simulink model "AEB_System"  (R2023a)
settings: Solver=FixedStepAuto  StartTime=0.0  StopTime=10.0  FixedStep=1  RelTol=1e-3
values from neighbouring files (symbols this model uses):
  AEB_Brake_Apply = 1.0    [AEB_Data.sldd]
  AEB_Warning = 1.0    [AEB_Data.sldd]
  Friction = 0.7    [AEB_Data.sldd]
  Gravity = 9.81    [AEB_Data.sldd]
  Growth_Time_Dec = 0.1    [AEB_Data.sldd]
  L_Limit = -1.1    [AEB_Data.sldd]
  Min_Dis_Stop_Veh = 2.0    [AEB_Data.sldd]
  No_Warning = 0.0    [AEB_Data.sldd]
  On_Value = 1.0    [AEB_Data.sldd]
  Out_Rang = 300.0    [AEB_Data.sldd]
  R_Limit = 1.1    [AEB_Data.sldd]
  Reac_Time = 1.0    [AEB_Data.sldd]
settings Model: DataDictionary=AEB_Data.sldd  Creator=songi  LastModifiedBy=songi
settings DebuggingCC: ParameterPrecisionLossMsg=none  UnitsInconsistencyMsg=none

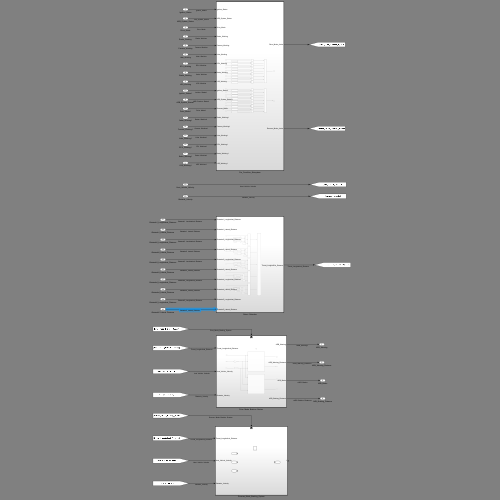
[thumbnail: Simulink's stored preview of the top-level diagram]
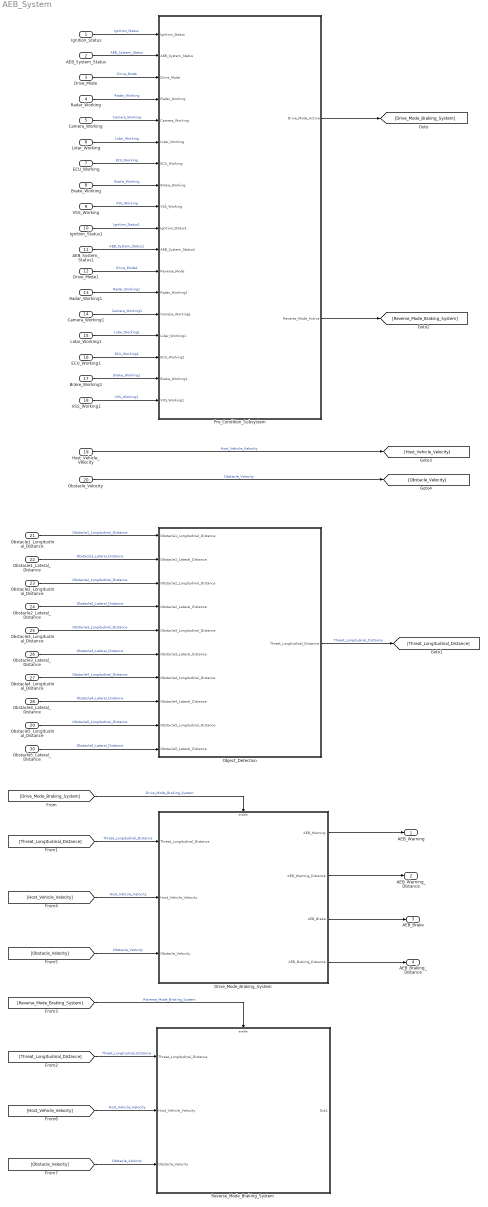
== system AEB_System ==
  Ignition_Status : Inport
  AEB_System_Status : Inport  Port=2
  Drive_Mode : Inport  Port=3
  Radar_Working : Inport  Port=4
  Camera_Working : Inport  Port=5
  Lidar_Working : Inport  Port=6
  ECU_Working : Inport  Port=7
  Brake_Working : Inport  Port=8
  VSS_Working : Inport  Port=9
  Ignition_Status1 : Inport  Port=10
  AEB_System_Status1 : Inport  Port=11
  Drive_Mode1 : Inport  Port=12
  Radar_Working1 : Inport  Port=13
  Camera_Working1 : Inport  Port=14
  Lidar_Working1 : Inport  Port=15
  ECU_Working1 : Inport  Port=16
  Brake_Working1 : Inport  Port=17
  VSS_Working1 : Inport  Port=18
  Host_Vehicle_Velocity : Inport  Port=19
  Obstacle_Velocity : Inport  Port=20
  Obstacle1_Longitudinal_Distance : Inport  Port=21
  Obstacle1_Lateral_Distance : Inport  Port=22
  Obstacle2_Longitudinal_Distance : Inport  Port=23
  Obstacle2_Lateral_Distance : Inport  Port=24
  Obstacle3_Longitudinal_Distance : Inport  Port=25
  Obstacle3_Lateral_Distance : Inport  Port=26
  Obstacle4_Longitudinal_Distance : Inport  Port=27
  Obstacle4_Lateral_Distance : Inport  Port=28
  Obstacle5_Longitudinal_Distance : Inport  Port=29
  Obstacle5_Lateral_Distance : Inport  Port=30
  Drive_Mode_Braking_System : Subsystem  TreatAsAtomicUnit=on
  Object_Detection : Subsystem  TreatAsAtomicUnit=on
  Pre_Condition_Subsystem : Subsystem  TreatAsAtomicUnit=on
  Reverse_Mode_Braking_System : Subsystem  TreatAsAtomicUnit=on
  AEB_Warning : Outport
  AEB_Warning_Distance : Outport  Port=2
  AEB_Brake : Outport  Port=3
  AEB_Braking_Distance : Outport  Port=4
  wires:
  Ignition_Status/1 -> Pre_Condition_Subsystem/1(Ignition_Status)  "Ignition_Status"
  AEB_System_Status/1 -> Pre_Condition_Subsystem/2(AEB_System_Status)  "AEB_System_Status"
  Drive_Mode/1 -> Pre_Condition_Subsystem/3(Drive_Mode)  "Drive_Mode"
  Radar_Working/1 -> Pre_Condition_Subsystem/4(Radar_Working)  "Radar_Working"
  Camera_Working/1 -> Pre_Condition_Subsystem/5(Camera_Working)  "Camera_Working"
  Lidar_Working/1 -> Pre_Condition_Subsystem/6(Lidar_Working)  "Lidar_Working"
  ECU_Working/1 -> Pre_Condition_Subsystem/7(ECU_Working)  "ECU_Working"
  Brake_Working/1 -> Pre_Condition_Subsystem/8(Brake_Working)  "Brake_Working"
  VSS_Working/1 -> Pre_Condition_Subsystem/9(VSS_Working)  "VSS_Working"
  Obstacle2_Longitudinal_Distance/1 -> Object_Detection/3(Obstacle2_Longitudinal_Distance)  "Obstacle2_Longitudinal_Distance"
  Obstacle2_Lateral_Distance/1 -> Object_Detection/4(Obstacle2_Lateral_Distance)  "Obstacle2_Lateral_Distance"
  Obstacle3_Longitudinal_Distance/1 -> Object_Detection/5(Obstacle3_Longitudinal_Distance)  "Obstacle3_Longitudinal_Distance"
  Obstacle3_Lateral_Distance/1 -> Object_Detection/6(Obstacle3_Lateral_Distance)  "Obstacle3_Lateral_Distance"
  Obstacle4_Longitudinal_Distance/1 -> Object_Detection/7(Obstacle4_Longitudinal_Distance)  "Obstacle4_Longitudinal_Distance"
  Obstacle4_Lateral_Distance/1 -> Object_Detection/8(Obstacle4_Lateral_Distance)  "Obstacle4_Lateral_Distance"
  Obstacle5_Longitudinal_Distance/1 -> Object_Detection/9(Obstacle5_Longitudinal_Distance)  "Obstacle5_Longitudinal_Distance"
  Obstacle5_Lateral_Distance/1 -> Object_Detection/10(Obstacle5_Lateral_Distance)  "Obstacle5_Lateral_Distance"
  Pre_Condition_Subsystem/1(Drive_Mode_Active) -> [Drive_Mode_Braking_System]
  Pre_Condition_Subsystem/2(Reverse_Mode_Active) -> [Reverse_Mode_Braking_System]
  Ignition_Status1/1 -> Pre_Condition_Subsystem/10(Ignition_Status1)  "Ignition_Status1"
  VSS_Working1/1 -> Pre_Condition_Subsystem/18(VSS_Working1)  "VSS_Working1"
  AEB_System_Status1/1 -> Pre_Condition_Subsystem/11(AEB_System_Status1)  "AEB_System_Status1"
  Drive_Mode1/1 -> Pre_Condition_Subsystem/12(Reverse_Mode)  "Drive_Mode1"
  Radar_Working1/1 -> Pre_Condition_Subsystem/13(Radar_Working1)  "Radar_Working1"
  Camera_Working1/1 -> Pre_Condition_Subsystem/14(Camera_Working1)  "Camera_Working1"
  ECU_Working1/1 -> Pre_Condition_Subsystem/16(ECU_Working1)  "ECU_Working1"
  Lidar_Working1/1 -> Pre_Condition_Subsystem/15(Lidar_Working1)  "Lidar_Working1"
  Brake_Working1/1 -> Pre_Condition_Subsystem/17(Brake_Working1)  "Brake_Working1"
  Object_Detection/1(Threat_Longitudinal_Distance) -> [Threat_Longitudinal_Distance]  "Threat_Longitudinal_Distance"
  Host_Vehicle_Velocity/1 -> [Host_Vehicle_Velocity]  "Host_Vehicle_Velocity"
  Obstacle1_Longitudinal_Distance/1 -> Object_Detection/1(Obstacle1_Longitudinal_Distance)  "Obstacle1_Longitudinal_Distance"
  Obstacle1_Lateral_Distance/1 -> Object_Detection/2(Obstacle1_Lateral_Distance)  "Obstacle1_Lateral_Distance"
  Obstacle_Velocity/1 -> [Obstacle_Velocity]  "Obstacle_Velocity"
  [Threat_Longitudinal_Distance] -> Drive_Mode_Braking_System/1(Threat_Longitudinal_Distance)  "Threat_Longitudinal_Distance"
  [Obstacle_Velocity] -> Drive_Mode_Braking_System/3(Obstacle_Velocity)  "Obstacle_Velocity"
  [Reverse_Mode_Braking_System] -> Reverse_Mode_Braking_System/Enable  "Reverse_Mode_Braking_System"
  [Obstacle_Velocity] -> Reverse_Mode_Braking_System/3(Obstacle_Velocity)  "Obstacle_Velocity"
  [Threat_Longitudinal_Distance] -> Reverse_Mode_Braking_System/1(Threat_Longitudinal_Distance)  "Threat_Longitudinal_Distance"
  [Drive_Mode_Braking_System] -> Drive_Mode_Braking_System/Enable  "Drive_Mode_Braking_System"
  [Host_Vehicle_Velocity] -> Reverse_Mode_Braking_System/2(Host_Vehicle_Velocity)  "Host_Vehicle_Velocity"
  Drive_Mode_Braking_System/1(AEB_Warning) -> AEB_Warning/1
  Drive_Mode_Braking_System/2(AEB_Warning_Distance) -> AEB_Warning_Distance/1
  Drive_Mode_Braking_System/3(AEB_Brake) -> AEB_Brake/1
  Drive_Mode_Braking_System/4(AEB_Braking_Distance) -> AEB_Braking_Distance/1
  [Host_Vehicle_Velocity] -> Drive_Mode_Braking_System/2(Host_Vehicle_Velocity)  "Host_Vehicle_Velocity"

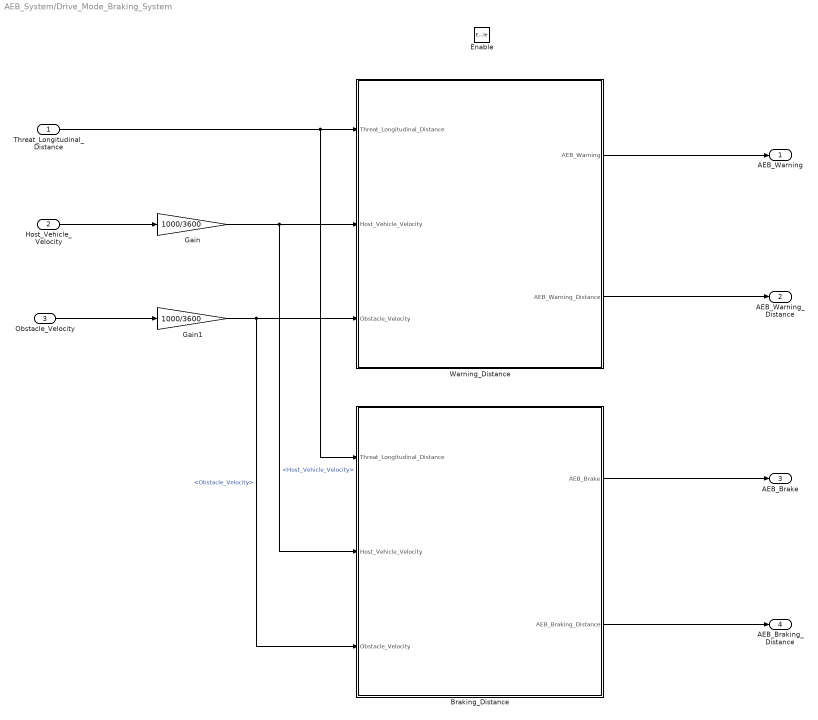
== system AEB_System/Drive_Mode_Braking_System ==
  Threat_Longitudinal_Distance : Inport
  Host_Vehicle_Velocity : Inport  Port=2
  Obstacle_Velocity : Inport  Port=3
  Enable : EnablePort
  Braking_Distance : Subsystem  TreatAsAtomicUnit=on
  Gain : Gain  Gain=1000/3600  OutDataTypeStr=half
  Gain1 : Gain  Gain=1000/3600  OutDataTypeStr=half
  Warning_Distance : Subsystem  TreatAsAtomicUnit=on
  AEB_Warning : Outport
  AEB_Warning_Distance : Outport  Port=2
  AEB_Brake : Outport  Port=3
  AEB_Braking_Distance : Outport  Port=4
  wires:
  Threat_Longitudinal_Distance/1 -> Braking_Distance/1(Threat_Longitudinal_Distance), Warning_Distance/1(Threat_Longitudinal_Distance)
  Warning_Distance/1(AEB_Warning) -> AEB_Warning/1
  Warning_Distance/2(AEB_Warning_Distance) -> AEB_Warning_Distance/1
  Braking_Distance/1(AEB_Brake) -> AEB_Brake/1
  Braking_Distance/2(AEB_Braking_Distance) -> AEB_Braking_Distance/1
  Obstacle_Velocity/1 -> Gain1/1
  Gain1/1 -> Braking_Distance/3(Obstacle_Velocity), Warning_Distance/3(Obstacle_Velocity)  "<Obstacle_Velocity>"
  Host_Vehicle_Velocity/1 -> Gain/1
  Gain/1 -> Braking_Distance/2(Host_Vehicle_Velocity), Warning_Distance/2(Host_Vehicle_Velocity)  "<Host_Vehicle_Velocity>"

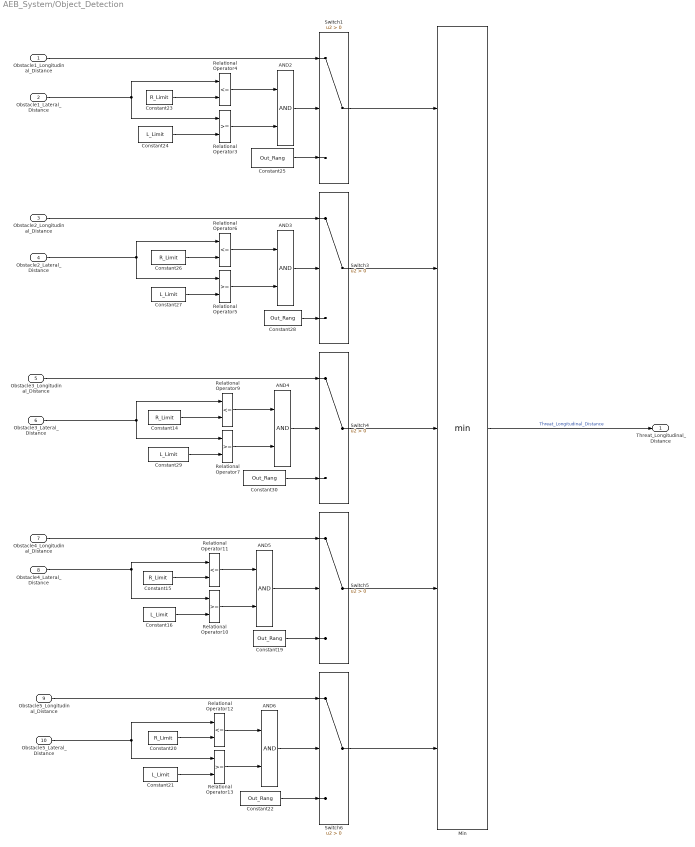
== system AEB_System/Object_Detection ==
  Obstacle1_Longitudinal_Distance : Inport
  Obstacle1_Lateral_Distance : Inport  Port=2
  Obstacle2_Longitudinal_Distance : Inport  Port=3
  Obstacle2_Lateral_Distance : Inport  Port=4
  Obstacle3_Longitudinal_Distance : Inport  Port=5
  Obstacle3_Lateral_Distance : Inport  Port=6
  Obstacle4_Longitudinal_Distance : Inport  Port=7
  Obstacle4_Lateral_Distance : Inport  Port=8
  Obstacle5_Longitudinal_Distance : Inport  Port=9
  Obstacle5_Lateral_Distance : Inport  Port=10
  AND{2..6} (5 alike) : Logic  AllPortsSameDT=off  OutDataTypeStr=boolean
  Constant{14..15,20,23,26} (5 alike) : Constant  Value=R_Limit
  Constant{16,21,24,27,29} (5 alike) : Constant  Value=L_Limit
  Constant{19,22,25,28,30} (5 alike) : Constant  Value=Out_Rang
  Min : MinMax  Inputs=5
  Relational Operator{3,5,7,10,13} (5 alike) : RelationalOperator  OutDataTypeStr=boolean  RndMeth=Simplest  InputSameDT=off
  Relational Operator{4,6,9,11..12} (5 alike) : RelationalOperator  Operator=<=  OutDataTypeStr=boolean  RndMeth=Simplest  InputSameDT=off
  Switch{1,3..6} (5 alike) : Switch  Criteria=u2 > Threshold  SaturateOnIntegerOverflow=off  InputSameDT=off
  Threat_Longitudinal_Distance : Outport
  wires:
  AND5/1 -> Switch5/2
  Relational Operator12/1 -> AND6/1
  Constant25/1 -> Switch1/3
  Relational Operator13/1 -> AND6/2
  Constant30/1 -> Switch4/3
  Constant21/1 -> Relational Operator13/2
  Constant15/1 -> Relational Operator11/2
  Constant29/1 -> Relational Operator7/2
  AND3/1 -> Switch3/2
  Relational Operator11/1 -> AND5/1
  Obstacle2_Lateral_Distance/1 -> Relational Operator5/1, Relational Operator6/1
  Obstacle1_Longitudinal_Distance/1 -> Switch1/1
  Obstacle5_Longitudinal_Distance/1 -> Switch6/1
  Min/1 -> Threat_Longitudinal_Distance/1  "Threat_Longitudinal_Distance"
  Switch3/1 -> Min/2
  Relational Operator4/1 -> AND2/1
  Relational Operator7/1 -> AND4/2
  Obstacle3_Lateral_Distance/1 -> Relational Operator7/1, Relational Operator9/1
  Relational Operator3/1 -> AND2/2
  Constant27/1 -> Relational Operator5/2
  Relational Operator5/1 -> AND3/2
  AND2/1 -> Switch1/2
  Switch4/1 -> Min/3
  Relational Operator10/1 -> AND5/2
  AND4/1 -> Switch4/2
  Relational Operator6/1 -> AND3/1
  Constant23/1 -> Relational Operator4/2
  Switch1/1 -> Min/1
  Obstacle5_Lateral_Distance/1 -> Relational Operator13/1, Relational Operator12/1
  Obstacle2_Longitudinal_Distance/1 -> Switch3/1
  Constant20/1 -> Relational Operator12/2
  Obstacle1_Lateral_Distance/1 -> Relational Operator4/1, Relational Operator3/1
  Switch5/1 -> Min/4
  Obstacle4_Longitudinal_Distance/1 -> Switch5/1
  AND6/1 -> Switch6/2
  Constant28/1 -> Switch3/3
  Constant26/1 -> Relational Operator6/2
  Constant16/1 -> Relational Operator10/2
  Constant22/1 -> Switch6/3
  Obstacle4_Lateral_Distance/1 -> Relational Operator11/1, Relational Operator10/1
  Relational Operator9/1 -> AND4/1
  Switch6/1 -> Min/5
  Constant24/1 -> Relational Operator3/2
  Constant14/1 -> Relational Operator9/2
  Constant19/1 -> Switch5/3
  Obstacle3_Longitudinal_Distance/1 -> Switch4/1

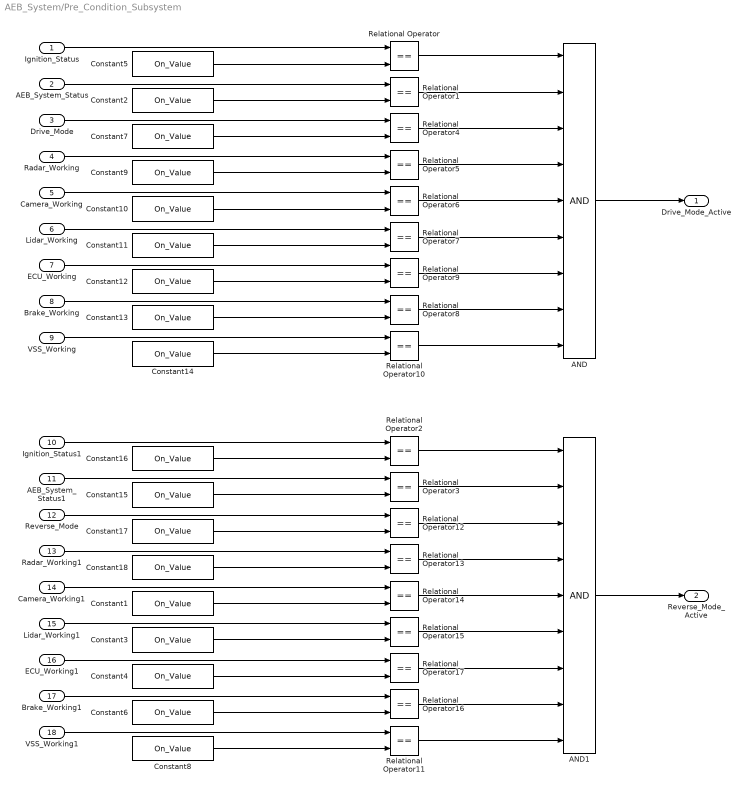
== system AEB_System/Pre_Condition_Subsystem ==
  Ignition_Status : Inport  OutDataTypeStr=boolean
  AEB_System_Status : Inport  Port=2  OutDataTypeStr=boolean
  Drive_Mode : Inport  Port=3  OutDataTypeStr=boolean
  Radar_Working : Inport  Port=4  OutDataTypeStr=boolean
  Camera_Working : Inport  Port=5  OutDataTypeStr=boolean
  Lidar_Working : Inport  Port=6  OutDataTypeStr=boolean
  ECU_Working : Inport  Port=7  OutDataTypeStr=boolean
  Brake_Working : Inport  Port=8  OutDataTypeStr=boolean
  VSS_Working : Inport  Port=9  OutDataTypeStr=boolean
  Ignition_Status1 : Inport  Port=10  OutDataTypeStr=boolean
  AEB_System_Status1 : Inport  Port=11  OutDataTypeStr=boolean
  Reverse_Mode : Inport  Port=12  OutDataTypeStr=boolean
  Radar_Working1 : Inport  Port=13  OutDataTypeStr=boolean
  Camera_Working1 : Inport  Port=14  OutDataTypeStr=boolean
  Lidar_Working1 : Inport  Port=15  OutDataTypeStr=boolean
  ECU_Working1 : Inport  Port=16  OutDataTypeStr=boolean
  Brake_Working1 : Inport  Port=17  OutDataTypeStr=boolean
  VSS_Working1 : Inport  Port=18  OutDataTypeStr=boolean
  AND : Logic  Inputs=9  AllPortsSameDT=off  OutDataTypeStr=boolean
  AND1 : Logic  Inputs=9  AllPortsSameDT=off  OutDataTypeStr=boolean
  Constant{1..18} (18 alike) : Constant  Value=On_Value
  Relational Operator{,1..17} (18 alike) : RelationalOperator  Operator===  OutDataTypeStr=boolean  RndMeth=Simplest  InputSameDT=off
  Drive_Mode_Active : Outport
  Reverse_Mode_Active : Outport  Port=2
  wires:
  Relational Operator/1 -> AND/1
  Relational Operator1/1 -> AND/2
  AEB_System_Status/1 -> Relational Operator1/1
  Ignition_Status/1 -> Relational Operator/1
  Constant5/1 -> Relational Operator/2
  Constant2/1 -> Relational Operator1/2
  Drive_Mode/1 -> Relational Operator4/1
  Constant7/1 -> Relational Operator4/2
  AND/1 -> Drive_Mode_Active/1
  Lidar_Working/1 -> Relational Operator7/1
  Brake_Working/1 -> Relational Operator8/1
  Constant12/1 -> Relational Operator9/2
  ECU_Working/1 -> Relational Operator9/1
  Constant11/1 -> Relational Operator7/2
  Constant13/1 -> Relational Operator8/2
  Constant10/1 -> Relational Operator6/2
  Constant9/1 -> Relational Operator5/2
  Radar_Working/1 -> Relational Operator5/1
  Camera_Working/1 -> Relational Operator6/1
  Constant14/1 -> Relational Operator10/2
  VSS_Working/1 -> Relational Operator10/1
  Relational Operator4/1 -> AND/3
  Relational Operator5/1 -> AND/4
  Relational Operator6/1 -> AND/5
  Relational Operator7/1 -> AND/6
  Relational Operator9/1 -> AND/7
  Relational Operator8/1 -> AND/8
  Relational Operator10/1 -> AND/9
  Relational Operator17/1 -> AND1/7
  Relational Operator15/1 -> AND1/6
  Ignition_Status1/1 -> Relational Operator2/1
  VSS_Working1/1 -> Relational Operator11/1
  ECU_Working1/1 -> Relational Operator17/1
  Constant6/1 -> Relational Operator16/2
  Brake_Working1/1 -> Relational Operator16/1
  Constant4/1 -> Relational Operator17/2
  Constant17/1 -> Relational Operator12/2
  Relational Operator16/1 -> AND1/8
  Constant3/1 -> Relational Operator15/2
  Constant1/1 -> Relational Operator14/2
  Relational Operator3/1 -> AND1/2
  Constant8/1 -> Relational Operator11/2
  AEB_System_Status1/1 -> Relational Operator3/1
  Relational Operator13/1 -> AND1/4
  AND1/1 -> Reverse_Mode_Active/1
  Lidar_Working1/1 -> Relational Operator15/1
  Reverse_Mode/1 -> Relational Operator12/1
  Constant15/1 -> Relational Operator3/2
  Camera_Working1/1 -> Relational Operator14/1
  Radar_Working1/1 -> Relational Operator13/1
  Relational Operator2/1 -> AND1/1
  Constant16/1 -> Relational Operator2/2
  Relational Operator12/1 -> AND1/3
  Relational Operator11/1 -> AND1/9
  Relational Operator14/1 -> AND1/5
  Constant18/1 -> Relational Operator13/2

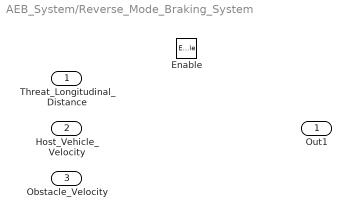
== system AEB_System/Reverse_Mode_Braking_System ==
  Threat_Longitudinal_Distance : Inport
  Host_Vehicle_Velocity : Inport  Port=2
  Obstacle_Velocity : Inport  Port=3
  Enable : EnablePort
  Out1 : Outport

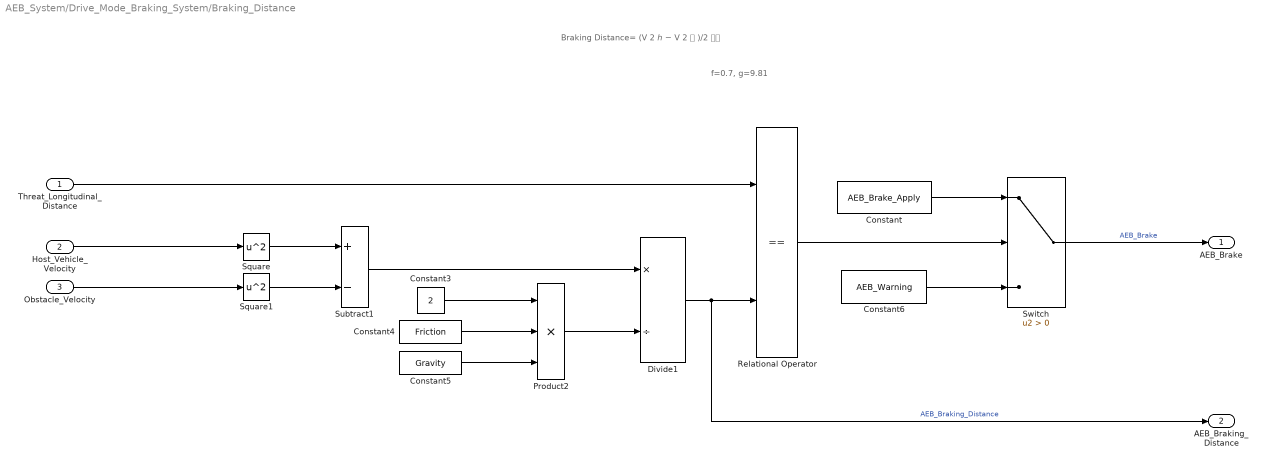
== system AEB_System/Drive_Mode_Braking_System/Braking_Distance ==
  note: Braking Distance= (V 2 ℎ − V 2 𝑙 )/2 𝑓𝑔
  note: f=0.7, g=9.81
  Threat_Longitudinal_Distance : Inport
  Host_Vehicle_Velocity : Inport  Port=2
  Obstacle_Velocity : Inport  Port=3
  Constant : Constant  Value=AEB_Brake_Apply
  Constant3 : Constant  Value=2
  Constant4 : Constant  Value=Friction
  Constant5 : Constant  Value=Gravity
  Constant6 : Constant  Value=AEB_Warning
  Divide1 : Product  Inputs=*/
  Product2 : Product  Inputs=3
  Relational Operator : RelationalOperator  Operator===  OutDataTypeStr=boolean  RndMeth=Simplest  InputSameDT=off
  Square : Math  Operator=square
  Square1 : Math  Operator=square
  Subtract1 : Sum  Inputs=+-
  Switch : Switch  Criteria=u2 > Threshold  SaturateOnIntegerOverflow=off  InputSameDT=off
  AEB_Brake : Outport
  AEB_Braking_Distance : Outport  Port=2
  wires:
  Constant5/1 -> Product2/3
  Square/1 -> Subtract1/1
  Subtract1/1 -> Divide1/1
  Square1/1 -> Subtract1/2
  Constant3/1 -> Product2/1
  Product2/1 -> Divide1/2
  Host_Vehicle_Velocity/1 -> Square/1
  Obstacle_Velocity/1 -> Square1/1
  Constant4/1 -> Product2/2
  Threat_Longitudinal_Distance/1 -> Relational Operator/1
  Relational Operator/1 -> Switch/2
  Switch/1 -> AEB_Brake/1  "AEB_Brake"
  Constant/1 -> Switch/1
  Constant6/1 -> Switch/3
  Divide1/1 -> Relational Operator/2, AEB_Braking_Distance/1  "AEB_Braking_Distance"

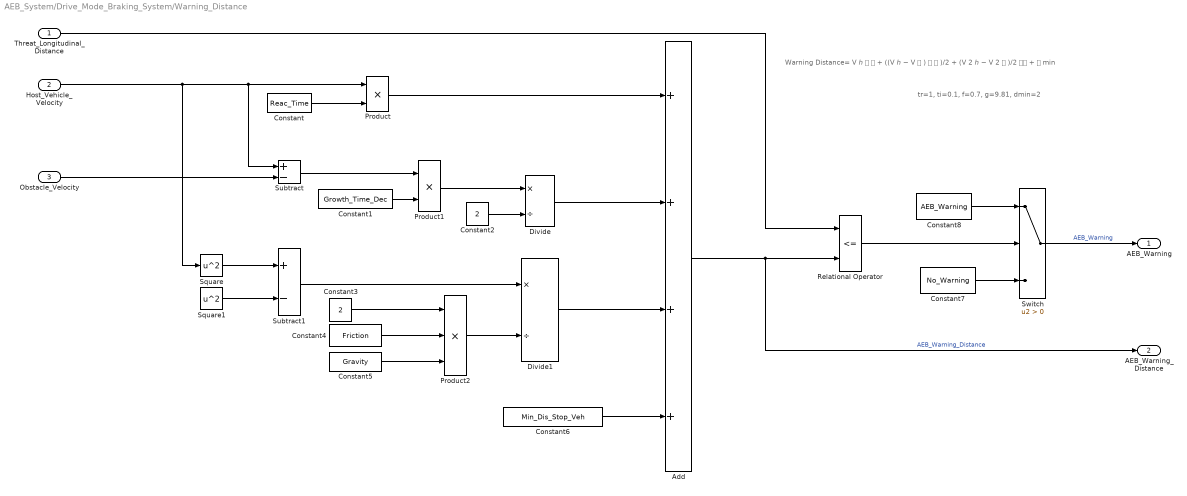
== system AEB_System/Drive_Mode_Braking_System/Warning_Distance ==
  note: tr=1, ti=0.1, f=0.7, g=9.81, dmin=2
  note: Warning Distance= V ℎ 𝑡 𝑟 + ((V ℎ − V 𝑙 ) 𝑡 𝑖 )/2 + (V 2 ℎ − V 2 𝑙 )/2 𝑓𝑔 + 𝑑 min
  Threat_Longitudinal_Distance : Inport
  Host_Vehicle_Velocity : Inport  Port=2
  Obstacle_Velocity : Inport  Port=3
  Add : Sum  Inputs=++++
  Constant : Constant  Value=Reac_Time
  Constant1 : Constant  Value=Growth_Time_Dec
  Constant2 : Constant  Value=2
  Constant3 : Constant  Value=2
  Constant4 : Constant  Value=Friction
  Constant5 : Constant  Value=Gravity
  Constant6 : Constant  Value=Min_Dis_Stop_Veh
  Constant7 : Constant  Value=No_Warning
  Constant8 : Constant  Value=AEB_Warning
  Divide : Product  Inputs=*/
  Divide1 : Product  Inputs=*/
  Product : Product
  Product1 : Product
  Product2 : Product  Inputs=3
  Relational Operator : RelationalOperator  Operator=<=  OutDataTypeStr=boolean  RndMeth=Simplest  InputSameDT=off
  Square : Math  Operator=square
  Square1 : Math  Operator=square
  Subtract : Sum  Inputs=+-
  Subtract1 : Sum  Inputs=+-
  Switch : Switch  Criteria=u2 > Threshold  SaturateOnIntegerOverflow=off  InputSameDT=off
  AEB_Warning : Outport
  AEB_Warning_Distance : Outport  Port=2
  wires:
  Constant7/1 -> Switch/3
  Constant2/1 -> Divide/2
  Constant4/1 -> Product2/2
  Host_Vehicle_Velocity/1 -> Subtract/1, Product/1, Square/1
  Product/1 -> Add/1
  Add/1 -> Relational Operator/2, AEB_Warning_Distance/1  "AEB_Warning_Distance"
  Divide1/1 -> Add/3
  Divide/1 -> Add/2
  Constant8/1 -> Switch/1
  Product2/1 -> Divide1/2
  Product1/1 -> Divide/1
  Constant/1 -> Product/2
  Constant3/1 -> Product2/1
  Square1/1 -> Subtract1/2
  Constant1/1 -> Product1/2
  Constant6/1 -> Add/4
  Subtract1/1 -> Divide1/1
  Square/1 -> Subtract1/1
  Constant5/1 -> Product2/3
  Subtract/1 -> Product1/1
  Threat_Longitudinal_Distance/1 -> Relational Operator/1
  Relational Operator/1 -> Switch/2
  Switch/1 -> AEB_Warning/1  "AEB_Warning"
  Obstacle_Velocity/1 -> Subtract/2
